simulink model "SEA_position_control"  (R2021a)
settings: Solver=ode4  StartTime=0.0  StopTime=50  FixedStep=0.0001  RelTol=1e-3
InitFcn:
  | Im=1;
  | Ij=0.1;
  | k_s=3000;
  | r=0.015;
  | Bm = 0.3;
  | Bj = 0.1;
  | wc = 100 ;
values from neighbouring files (symbols this model uses):
  s = tf('s')    [SEA_stiffness_selection_paper_derivation.m]    (also in mgridtesting.m)
libraries: dspstat3 x2, slctrlblks x1, pid_lib x1
settings Model: Creator=aarti  LastModifiedBy=Riswadkar

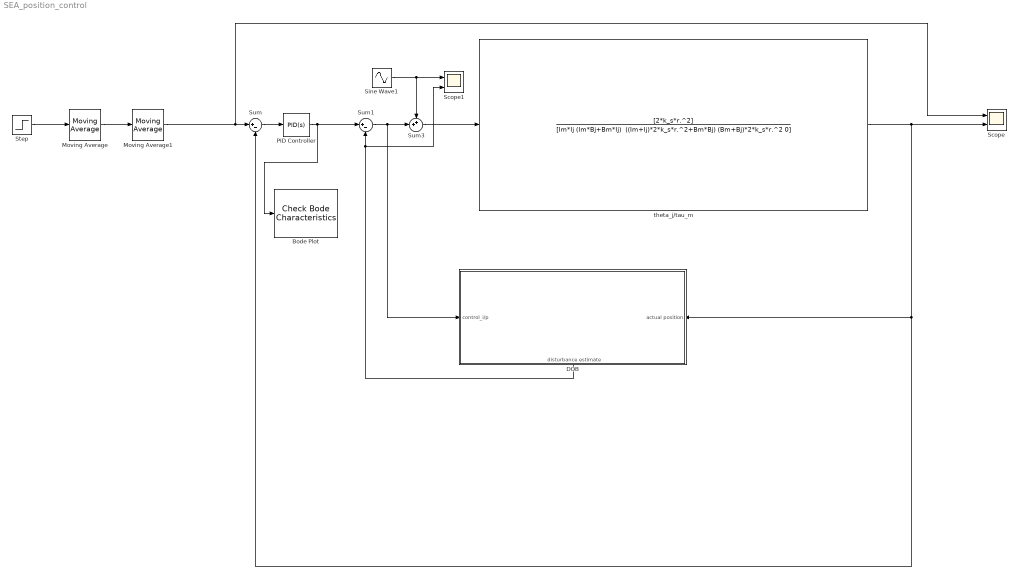
== system SEA_position_control ==
  Bode Plot : slctrlblks/Model Verification/Check Bode  Characteristics  InstantiateOnLoad=on  SaveOperatingPoints=off  LinearizationIOs={'/PID Controller', 1, 'in', 'off', '';'/theta_j//tau_m', 1, 'out', 'off', ''}  LinearizeAt=ExternalTrigger  SnapshotTimes=[0]  TriggerType=rising  SampleTime=auto  RateConversionMethod=zoh  PreWarpFreq=10  UseExactDelayModel=off  UseFullBlockNameLabels=off  UseBusSignalLabels=off  enabled=on  stopWhenAssertionFail=off  export=off  ViewDlgPos=[642.6 79.4 509.6 389.6]  OpenViewOnLoad=off  LaunchViewOnOpen=off  FrequencyUnits=rad/s  MagnitudeUnits=dB  PhaseUnits=deg  TimeUnits=seconds  EnableUpperBound=off  UpperBoundFrequencies=[]  UpperBoundMagnitudes=[]  EnableLowerBound=off  LowerBoundFrequencies=[]  LowerBoundMagnitudes=[]
  DOB : Subsystem
      settings: PortSchema="{\"entries\":[{\"content\":{\"sides\":[{\"content\":{\"connectorIds\":[\"In1\"]},\"type\":\"ConnectorPlacement.EquallySpacedRectSide\",\"uuid\":\"39ece9b6-474b-4a00-97b3-8efc39b44a1e\"},{\"content\":{\"connectorIds\":[\"In2\"],\"side\":\"RIGHT\"},\"type\":\"ConnectorPlacement.EquallySpacedRectSide\",\"uuid\":\"047ce420-0e52-454f-a43b-d37f0edecad8\"},{\"content\":{\"connectorIds\":[],\"side\":\"TOP\"},\"type\":\"ConnectorPlacement.EquallySpacedRectSide\",\"uuid\":\"5b6783e4-3108-4af7-83a7-5877d2ed5b46\"},{\"content\":{\"connectorIds\":[\"Out1\"],\"side\":\"BOTTOM\"},\"type\":\"ConnectorPlacement.EquallySpacedRectSide\",\"uuid\":\"7ca089e3-b282-4207-8701-312757589b4a\"}]},\"type\":\"ConnectorPlacement.EquallySpacedConnector\",\"uuid\":\"76d8437d-8186-41db-9f91-f938acbc2c7d\"}],\"packageUris\":[\"http://schema.mathworks.com/mf0/Connector/R2020b\"],\"version\":\"1.0\"}"
  Moving Average : dspstat3/Moving Average  Method=Sliding window  ForgettingFactorPort=off  SpecifyWindowLength=on  WindowLength=10000  ForgettingFactor=0.9  SimulateUsing=Code generation
  Moving Average1 : dspstat3/Moving Average  Method=Sliding window  ForgettingFactorPort=off  SpecifyWindowLength=on  WindowLength=10000  ForgettingFactor=0.9  SimulateUsing=Code generation
  PID Controller : pid_lib/PID Controller  Controller=PID  Form=Parallel  TimeDomain=Continuous-time  UseExternalTs=off  SampleTime=-1  IntegratorMethod=Forward Euler  FilterMethod=Forward Euler  ControllerParametersSource=internal  P=0.1  I=0.4  D=2  UseFilter=on  N=1.8  TunerSelectOption=Transfer Function Based (PID Tuner App)  InitialConditionSource=internal  InitialConditionForIntegrator=0  InitialConditionForFilter=0  DifferentiatorICPrevScaledInput=0  ExternalReset=none  TrackingMode=off  Kt=1  LimitOutput=off  SatLimitsSource=internal  UpperSaturationLimit=inf  LowerSaturationLimit=-inf  LinearizeAsGain=on  AntiWindupMode=none  Kb=1  POutMin=[]  POutMax=[]  IOutMin=[]  IOutMax=[]  DOutMin=[]  DOutMax=[]  NOutMin=[]  NOutMax=[]  SumOutMin=[]  SumOutMax=[]  SaturationOutMin=[]  SaturationOutMax=[]  PParamMin=[]  PParamMax=[]  IParamMin=[]  IParamMax=[]  DParamMin=[]  DParamMax=[]  NParamMin=[]  NParamMax=[]  KbParamMin=[]  KbParamMax=[]  KtParamMin=[]  KtParamMax=[]  KbOutMin=[]  KbOutMax=[]  KtOutMin=[]  KtOutMax=[]  IntegratorOutMin=[]  IntegratorOutMax=[]  FilterOutMin=[]  FilterOutMax=[]  SumI1OutMin=[]  SumI1OutMax=[]  SumI2OutMin=[]  SumI2OutMax=[]  SumI3OutMin=[]  SumI3OutMax=[]  SumI4OutMin=[]  SumI4OutMax=[]  SumDOutMin=[]  SumDOutMax=[]  DifferentiatorOutMin=[]  DifferentiatorOutMax=[]  FilterDiffOutCoefMin=[]  FilterDiffOutCoefMax=[]  ReciprocalOutMin=[]  ReciprocalOutMax=[]  SumDenOutMin=[]  SumDenOutMax=[]  SumNumOutMin=[]  SumNumOutMax=[]  DivideOutMin=[]  DivideOutMax=[]  UdiffTsProdOutMin=[]  UdiffTsProdOutMax=[]  NTsProdOutMin=[]  NTsProdOutMax=[]  UintegralTsProdOutMin=[]  UintegralTsProdOutMax=[]  UngainTsProdOutMin=[]  UngainTsProdOutMax=[]  IntegratorContinuousStateAttributes=''  IntegratorStateMustResolveToSignalObject=off  IntegratorRTWStateStorageClass=Auto  FilterContinuousStateAttributes=''  FilterStateMustResolveToSignalObject=off  FilterRTWStateStorageClass=Auto  ParallelPVariant=InternalParameters  IdealPVariant=Disabled  IVariant=InternalParameters  DVariant=InternalParameters  IntegratorVariant=Continuous  SatVariant=Disabled  AWVariant=Passthrough  PCopyVariant=Disabled  TRVariant=Disabled  FdbkBlocksVariant=Forward  IdealPFdbkVariant=Disabled  SatFdbkVariant=Disabled  DerivativeFilterVariant=ContFilter  NVariant=InternalParameters  NCopyVariant=Disabled  FilterICVariant=InternalICsFilter  IntegratorICVariant=InternalICs  ExternalResetVariant=Disabled  TRSumVariant=Passthrough  SumFdbkVariant=Disabled  SumVariant=Sum_PID  TsampFilterVariant=InternalTs  TsampNgainVariant=Passthrough  TsampIntegralVariant=Passthrough  ExternalSaturationOutDataTypeStr=Inherit: Same as second input
  Scope : Scope  NumInputPorts=2
  Scope1 : Scope  NumInputPorts=2
  Sine Wave1 : Sin  Frequency=50  SampleTime=0
  Step : Step  Time=5  SampleTime=0
  Sum : Sum  Inputs=|+-
  Sum1 : Sum  Inputs=|+-
  Sum3 : Sum  Inputs=++|
  theta_j/tau_m : TransferFcn  Numerator=[2*k_s*r.^2]  Denominator="[Im*Ij (Im*Bj+Bm*Ij)  ((Im+Ij)*2*k_s*r.^2+Bm*Bj) (Bm+Bj)*2*k_s*r.^2 0]"
  wires:
  Sum/1 -> PID Controller/1
  theta_j/tau_m/1 -> DOB/2(actual position), Sum/2, Scope/2
  Step/1 -> Moving Average/1
  Moving Average/1 -> Moving Average1/1
  PID Controller/1 -> Bode Plot/1, Sum1/1
  Sum3/1 -> theta_j/tau_m/1
  Sine Wave1/1 -> Sum3/1, Scope1/1
  Sum1/1 -> DOB/1(control_i/p), Sum3/2
  DOB/1(disturbance estimate) -> Scope1/2, Sum1/2
  Moving Average1/1 -> Scope/1, Sum/1

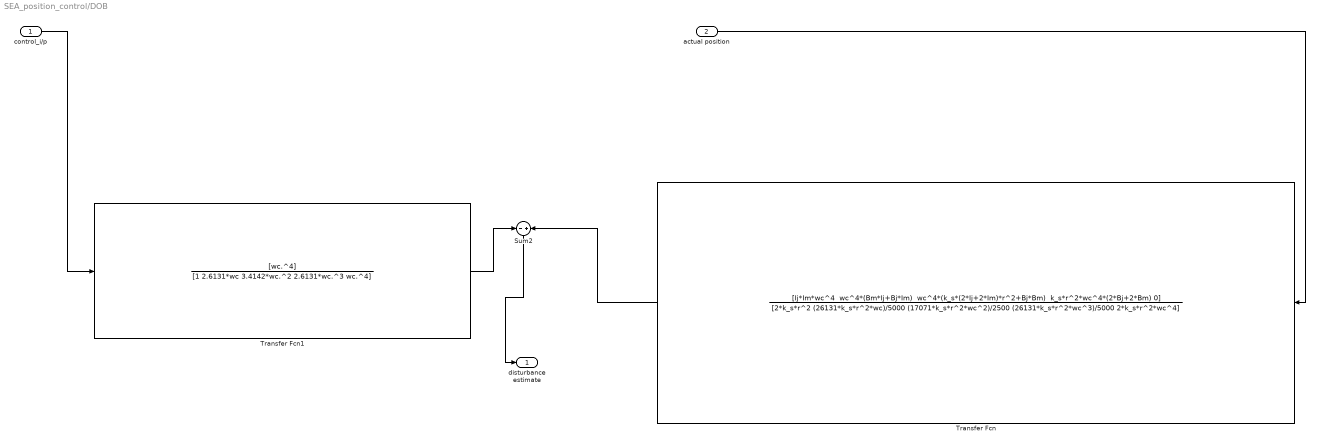
== system SEA_position_control/DOB ==
  control_i/p : Inport
  actual position : Inport  Port=2
  Sum2 : Sum  Inputs=-|+
  Transfer Fcn : TransferFcn  Numerator="[Ij*Im*wc^4  wc^4*(Bm*Ij+Bj*Im)  wc^4*(k_s*(2*Ij+2*Im)*r^2+Bj*Bm)  k_s*r^2*wc^4*(2*Bj+2*Bm) 0]"  Denominator=[2*k_s*r^2 (26131*k_s*r^2*wc)/5000 (17071*k_s*r^2*wc^2)/2500 (26131*k_s*r^2*wc^3)/5000 2*k_s*r^2*wc^4]
  Transfer Fcn1 : TransferFcn  Numerator=[wc.^4]  Denominator=[1 2.6131*wc 3.4142*wc.^2 2.6131*wc.^3 wc.^4]
  disturbance estimate : Outport
  wires:
  Transfer Fcn1/1 -> Sum2/1
  control_i/p/1 -> Transfer Fcn1/1
  Transfer Fcn/1 -> Sum2/2
  actual position/1 -> Transfer Fcn/1
  Sum2/1 -> disturbance estimate/1
